simulink subsystem "basic_infeed"  (R2023b)
settings: Solver=VariableStepAuto  StartTime=0.0  StopTime=10.0  RelTol=1e-3
model mask{P=0, Ts=0}
values from neighbouring files (symbols this model uses):
  Ts = ts(k)    [example_MW.m]
libraries: ee_lib x12, fl_lib x4, eeGeneralControl x3, nesl_utility x3, eeTransforms x2, eeSinusoidalMeasurement x1
settings Model: Creator=neugebch  LastModifiedBy=neugebch

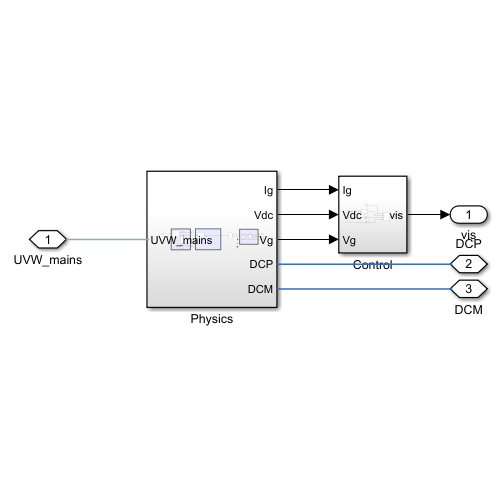
[thumbnail: Simulink's stored preview of the top-level diagram]
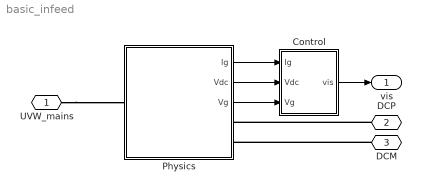
== system basic_infeed ==
  Control : Subsystem
  Physics : Subsystem
  UVW_mains : PMIOPort  Side=Left
  DCP : PMIOPort  Port=2  Side=Right
  DCM : PMIOPort  Port=3  Side=Right
  vis : Outport
  wires:
  Physics/3(Vg) -> Control/3(Vg)
  Physics/2(Vdc) -> Control/2(Vdc)
  Physics/1(Ig) -> Control/1(Ig)
  Control/1(vis) -> vis/1
  connections:
  DCM/RConn1 -- Physics/RConn2
  UVW_mains/RConn1 -- Physics/LConn1
  DCP/RConn1 -- Physics/RConn1

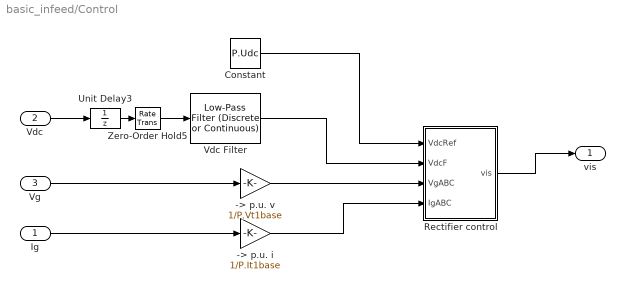
== system basic_infeed/Control ==
  Ig : Inport
  Vdc : Inport  Port=2
  Vg : Inport  Port=3
  -> p.u. i : Gain  Gain=1/P.It1base
  -> p.u. v : Gain  Gain=1/P.Vt1base
  Constant : Constant  Value=P.Udc
  Rectifier control : Subsystem
  Unit Delay3 : UnitDelay  SampleTime=Ts  HasFrameUpgradeWarning=on
  Vdc Filter : eeGeneralControl/Low-Pass Filter (Discrete or Continuous)  K=1  T=1e-3  B=inf  A=-inf  init_option=Inherited from block input  x0=0  Ts=P.Tsc
  Zero-Order Hold5 : RateTransition  OutPortSampleTime=5e-05
  vis : Outport
  wires:
  Zero-Order Hold5/1 -> Vdc Filter/1
  -> p.u. i/1 -> Rectifier control/4(IgABC)
  -> p.u. v/1 -> Rectifier control/3(VgABC)
  Vdc Filter/1 -> Rectifier control/2(VdcF)
  Unit Delay3/1 -> Zero-Order Hold5/1
  Vdc/1 -> Unit Delay3/1
  Constant/1 -> Rectifier control/1(VdcRef)
  Vg/1 -> -> p.u. v/1
  Rectifier control/1(vis) -> vis/1
  Ig/1 -> -> p.u. i/1

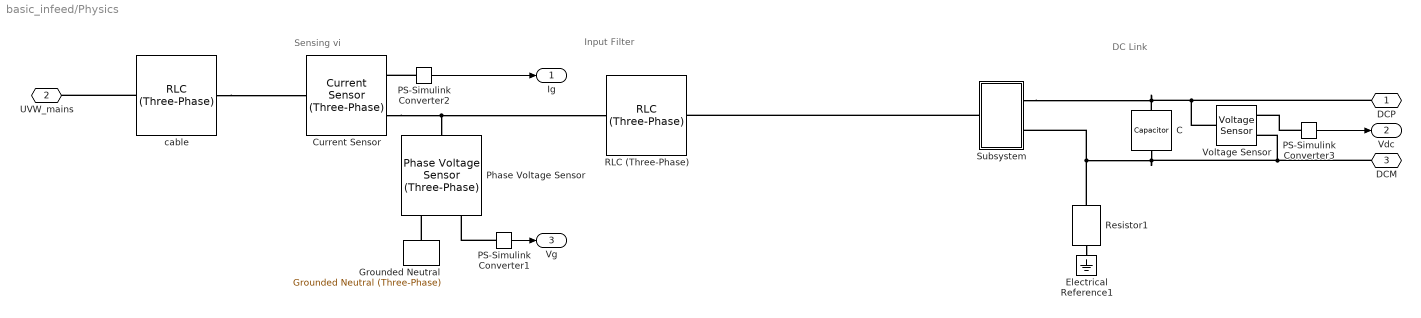
== system basic_infeed/Physics ==
  note: DC
      | Link
  note: Input Filter
  note: Sensing vi
  C : fl_lib/Electrical/Electrical Elements/Capacitor  c=P.Cd F  r=P.Rd Ohm  g=1/P.Rd2 1/Ohm  i_specify=off  i_priority=None  i=0 A  i_nominal_specify=off  i_nominal_unit=A  i_nominal_value=1  v_specify=off  v_priority=None  v=0 V  v_nominal_specify=off  v_nominal_unit=V  v_nominal_value=1  vc_specify=on  vc_priority=None  vc=0 V  vc_nominal_specify=off  vc_nominal_unit=V  vc_nominal_value=1
  Current Sensor : ee_lib/Sensors & Transducers/Current Sensor (Three-Phase)
  Electrical Reference1 : fl_lib/Electrical/Electrical Elements/Electrical Reference
  Grounded Neutral : ee_lib/Connectors & References/Grounded Neutral (Three-Phase)
  PS-Simulink Converter1 : nesl_utility/PS-Simulink Converter  PhysicalDomain=network_engine_domain  SubClassName=ps_output  LeftPortType=input  RightPortType=output  PseudoPeriodic=off  Frequencies=[]  VectorFormat=1-D array  Unit=1  AffineConversion=off
  PS-Simulink Converter2 : nesl_utility/PS-Simulink Converter  PhysicalDomain=network_engine_domain  SubClassName=ps_output  LeftPortType=input  RightPortType=output  PseudoPeriodic=off  Frequencies=[]  VectorFormat=1-D array  Unit=1  AffineConversion=off
  PS-Simulink Converter3 : nesl_utility/PS-Simulink Converter  PhysicalDomain=network_engine_domain  SubClassName=ps_output  LeftPortType=input  RightPortType=output  PseudoPeriodic=off  Frequencies=[]  VectorFormat=1-D array  Unit=1  AffineConversion=off
  Phase Voltage Sensor : ee_lib/Sensors & Transducers/Phase Voltage Sensor (Three-Phase)
  RLC (Three-Phase) : ee_lib/Passive/RLC Assemblies/RLC (Three-Phase)  component_structure=ee.enum.rlc.structure.SeriesRL  R=P.Lk*P.om/P.X_R_Lk Ohm  L=P.Lk H  C=1e-6 F  R_parasitic=0 Ohm  G_parasitic=0 1/Ohm  IL_specify=off  IL_priority=High  IL=[0, 0, 0] A  IL_nominal_specify=off  IL_nominal_unit=A  IL_nominal_value=1  VC_specify=off  VC_priority=High  VC=[0, 0, 0] V  VC_nominal_specify=off  VC_nominal_unit=V  VC_nominal_value=1
      settings: InternalSimscapePortConfiguration="{\"Bottom\":[],\"Left\":[{\"id\":\"N1\",\"label\":\"~1\",\"type\":\"foundation.electrical.three_phase\"}],\"Right\":[{\"id\":\"N2\",\"label\":\"~2\",\"type\":\"foundation.electrical.three_phase\"}],\"Top\":[]}"
  Resistor1 : fl_lib/Electrical/Electrical Elements/Resistor  R=1e5 Ohm  i_specify=off  i_priority=None  i=0 A  i_nominal_specify=off  i_nominal_unit=A  i_nominal_value=1  v_specify=off  v_priority=None  v=0 V  v_nominal_specify=off  v_nominal_unit=V  v_nominal_value=1
  Subsystem : Subsystem
  Voltage Sensor : fl_lib/Electrical/Electrical Sensors/Voltage Sensor
  cable : ee_lib/Passive/RLC Assemblies/RLC (Three-Phase)  component_structure=ee.enum.rlc.structure.SeriesRL  R=P.cab.l*P.cab.rl Ohm  L=P.cab.l*P.cab.ll H  C=1e-6 F  R_parasitic=0 Ohm  G_parasitic=0 1/Ohm  IL_specify=off  IL_priority=High  IL=[0, 0, 0] A  IL_nominal_specify=off  IL_nominal_unit=A  IL_nominal_value=1  VC_specify=off  VC_priority=High  VC=[0, 0, 0] V  VC_nominal_specify=off  VC_nominal_unit=V  VC_nominal_value=1
      settings: InternalSimscapePortConfiguration="{\"Bottom\":[],\"Left\":[{\"id\":\"N1\",\"label\":\"~1\",\"type\":\"foundation.electrical.three_phase\"}],\"Right\":[{\"id\":\"N2\",\"label\":\"~2\",\"type\":\"foundation.electrical.three_phase\"}],\"Top\":[]}"
  DCP : PMIOPort  Side=Right
  UVW_mains : PMIOPort  Port=2  Side=Left
  DCM : PMIOPort  Port=3  Side=Right
  Ig : Outport
  Vdc : Outport  Port=2
  Vg : Outport  Port=3
  wires:
  PS-Simulink Converter1/1 -> Vg/1
  PS-Simulink Converter2/1 -> Ig/1
  PS-Simulink Converter3/1 -> Vdc/1
  connections:
  cable/RConn1 -- Current Sensor/LConn1
  cable/LConn1 -- UVW_mains/RConn1
  Subsystem/LConn1 -- RLC (Three-Phase)/RConn1
  PS-Simulink Converter1/LConn1 -- Phase Voltage Sensor/RConn1
  Grounded Neutral/LConn1 -- Phase Voltage Sensor/RConn2
  Subsystem/RConn2 -- DCM/RConn1 -- Voltage Sensor/RConn2 -- C/RConn1 -- Resistor1/LConn1
  PS-Simulink Converter2/LConn1 -- Current Sensor/RConn1
  Current Sensor/RConn2 -- RLC (Three-Phase)/LConn1 -- Phase Voltage Sensor/LConn1
  C/LConn1 -- Subsystem/RConn1 -- Voltage Sensor/LConn1 -- DCP/RConn1
  PS-Simulink Converter3/LConn1 -- Voltage Sensor/RConn1
  Resistor1/RConn1 -- Electrical Reference1/LConn1

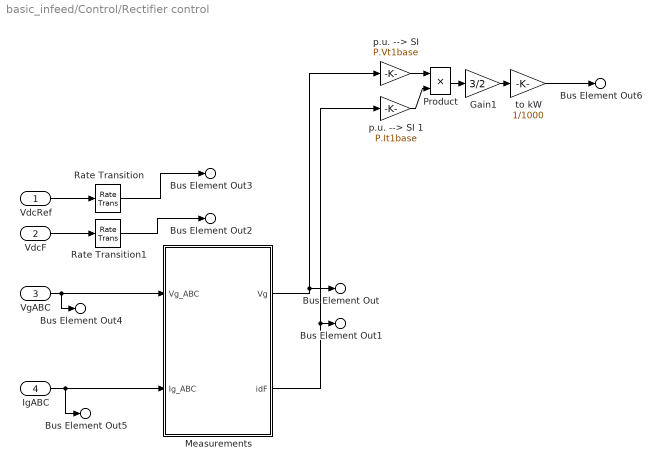
== system basic_infeed/Control/Rectifier control ==
  VdcRef : Inport
  VdcF : Inport  Port=2
  VgABC : Inport  Port=3
  IgABC : Inport  Port=4
  Gain1 : Gain  Gain=3/2
  Measurements : Subsystem
  Product : Product
  Rate Transition : RateTransition
  Rate Transition1 : RateTransition
  p.u. --> SI : Gain  Gain=P.Vt1base
  p.u. --> SI 1 : Gain  Gain=P.It1base
  to kW : Gain  Gain=1/1000
  Bus Element Out : Outport  PortName=vis  Element=Vg
  Bus Element Out1 : Outport  PortName=vis  Element=idF
  Bus Element Out2 : Outport  PortName=vis  Element=VdcF
  Bus Element Out3 : Outport  PortName=vis  Element=VdcRef
  Bus Element Out4 : Outport  PortName=vis  Element=VgABC
  Bus Element Out5 : Outport  PortName=vis  Element=IgABC
  Bus Element Out6 : Outport  PortName=vis  Element=Pt
  wires:
  VdcRef/1 -> Rate Transition/1
  VdcF/1 -> Rate Transition1/1
  VgABC/1 -> Bus Element Out4/1, Measurements/1(Vg_ABC)
  IgABC/1 -> Bus Element Out5/1, Measurements/2(Ig_ABC)
  Rate Transition/1 -> Bus Element Out3/1
  Rate Transition1/1 -> Bus Element Out2/1
  Measurements/1(Vg) -> p.u. --> SI/1, Bus Element Out/1
  Product/1 -> Gain1/1
  p.u. --> SI 1/1 -> Product/2
  p.u. --> SI/1 -> Product/1
  Gain1/1 -> to kW/1
  Measurements/2(idF) -> p.u. --> SI 1/1, Bus Element Out1/1
  to kW/1 -> Bus Element Out6/1

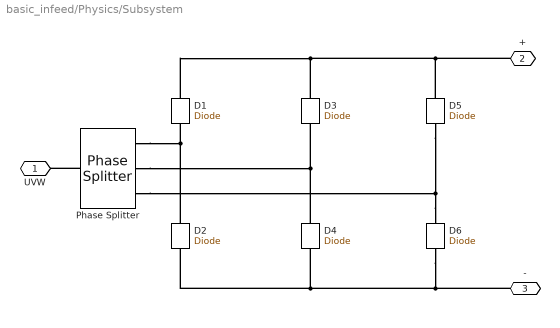
== system basic_infeed/Physics/Subsystem ==
  D{1..6} (6 alike) : ee_lib/Semiconductors & Converters/Diode  ModelType=ee.enum.diode.modelType.pwl  TableType=ee.enum.diode.tableType.IfMat  IfMat=[.07, .12, .19, 1.75, 4.24, 7.32, 11.2; .16, .3, .72, 2.14, 4.02, 6.35, 9.12] A  VfMat=[.9, 1.15, 1.25, 1.5, 1.75, 2.17, 2.6, 2.85; .58, .68, .75, 1.1, 1.38, 1.77, 2.27, 2.7] V  TjVec=[25, 125] degC  VfVec=[.5, .7, .9, 1.3, 1.7, 2.1, 2.5] V  IfVec=[.1, .2, .5, 1, 2, 4, 7, 10] A  Vf=0.6 V  Ron=0.3 Ohm  Goff=1e-8 S  prmExp=2  I12=[ 0.0137 0.545 ] A  V12=[ 0.6 0.7 ] V  RS=0.001 Ohm  Tmeas=25 degC  IS=1e-7 A  ec=1  I1=0.0137 A  V1=0.6 V  N_series=1  N_parallel=1  ZenerEnable=false  Rz=0.3 Ohm  BV=Inf V  C_param=1  CJ=50 pF  CJ0=50 pF  Vvec=[ 0.1 10 100 ] V  Cvec=[ 3.5 1 0.4 ] pF  VJ=1 V  Mgrad=0.5  FC=0.5  Q_param=ee.enum.diode.recoveryParam.off  iRM=-7.15 A  iF=4 A  didt=-750 A/us  trr_factor=3  trr=115 ns  Qrr=1500 s*uA  Vr=-600 V  Ls=150 nH  Erec=0.03 J  TT=50 ns  tau=100 ns  T_param=1  Tdevice=25 degC  I1_T2=0.245 A  V1_T2=0.5 V  IS_T2=1.25e-7 A  Tmeas2=125 degC  XTI_param=1  XTI=3  EG_param=1  EG=1.11 eV  dBVdT=0 V/K  enable_faults=ee.enum.enable.no  fault_action=simscape.enum.assert.action.none  fault_types=ee.enum.diode.faults.open  tau_fault=1e-3 s  IfMat_faulted=[.07, .12, .19, 1.75, 4.24, 7.32, 11.2; .16, .3, .72, 2.14, 4.02, 6.35, 9.12] A  VfMat_faulted=[.9, 1.15, 1.25, 1.5, 1.75, 2.17, 2.6, 2.85; .58, .68, .75, 1.1, 1.38, 1.77, 2.27, 2.7] V  VfVec_faulted=[.5, .7, .9, 1.3, 1.7, 2.1, 2.5] V  IfVec_faulted=[.1, .2, .5, 1, 2, 4, 7, 10] A  Ropen_faulted=1000 Ohm  Gshort_faulted=1000 1/Ohm  Vf_faulted=0.6 V  Ron_faulted=0.3 Ohm  Goff_faulted=1e-8 S  I12_faulted=[.0137, .545] A  V12_faulted=[.6, .7] V  IS_faulted=1e-12 A  ec_faulted=1  I1_faulted=0.0137 A  V1_faulted=0.6 V  RS_faulted=0 Ohm  Rz_faulted=0.3 Ohm  BV_faulted=inf V  Cscale_faulted=100  fault_trigger=ee.enum.faults.faultTrigger.temporal  t_fault=inf s  max_permissible_voltage=inf V  n_fail_on_voltage=1  max_permissible_current=inf A  t_fail_on_current=1 s  max_permissible_dVdt=inf V/s  enable_fault_input=simscape.enum.onoff.off  i_specify=off  i_priority=None  i=0 A  i_nominal_specify=off  i_nominal_unit=A  i_nominal_value=1  v_specify=off  v_priority=None  v=0 V  v_nominal_specify=off  v_nominal_unit=V  v_nominal_value=1  v_capacitor_specify=off  v_capacitor_priority=None  v_capacitor=0 V  v_capacitor_nominal_specify=off  v_capacitor_nominal_unit=V  v_capacitor_nominal_value=1  faulted_specify=off  faulted_priority=None  faulted=0  faulted_nominal_specify=off  faulted_nominal_unit=1  faulted_nominal_value=1  i_diode_specify=off  i_diode_priority=None  i_diode=0 A  i_diode_nominal_specify=off  i_diode_nominal_unit=A  i_diode_nominal_value=1  v_diode_specify=off  v_diode_priority=None  v_diode=0 V  v_diode_nominal_specify=off  v_diode_nominal_unit=V  v_diode_nominal_value=1  i_capacitor_specify=off  i_capacitor_priority=High  i_capacitor=0 A  i_capacitor_nominal_specify=off  i_capacitor_nominal_unit=A  i_capacitor_nominal_value=1  power_dissipated_specify=off  power_dissipated_priority=None  power_dissipated=0 W  power_dissipated_nominal_specify=off  power_dissipated_nominal_unit=W  power_dissipated_nominal_value=1  fidelity_level=ee.enum.diode.fidelity.includeChargeDyn  rec_loss_model=ee.enum.diode.reverseRecoveryModel.fixed  ErecVal=0 J  scaleWithIandV=true  ErecMat=zeros(2, 3) J  TjrecVec=[298.15, 398.15] K  IfrecVec=[.1, 1, 10] A  IrecVal=10 A  VrecVal=10 V  tFilter=1 / 1000 / 100 s  max_permissible_temperature=inf K  t_fail_on_temperature=1 s  thermal_network_parameterization=ee.enum.thermalNetworkTopology.junctionCase  Rth=[0, 10] K/W  Rth_Cauer=[1, 3, 10] K/W  Rth_Foster=[4, 6] K/W  thermal_mass_parameterization=ee.enum.thermalNetwork.timeconstant  thermal_mass=[0, 1] J/K  thermal_mass_Cauer=[.1, .3, 1] J/K  thermal_mass_Foster=[1.5, 3] J/K  thermal_time_constant=[0, 10] s  thermal_time_constant_Cauer=[1, 3, 10] s  thermal_time_constant_Foster=[6, 18] s  thermal_mass_initial_temperatures=[25, 25] degC  thermal_mass_initial_temperatures_Cauer=[25, 25, 25] degC  junction_thermal_mass=0.01 J/K  Tvec_initial_Foster=[25, 25, 25, 25] degC  no_thermal_network=0  junction_temperature_specify=off  junction_temperature_priority=None  junction_temperature=25 degC  junction_temperature_nominal_specify=off  junction_temperature_nominal_unit=degC  junction_temperature_nominal_value=1
      settings: LogSimulationData=on
  Phase Splitter : ee_lib/Connectors & References/Phase Splitter
  UVW : PMIOPort  Side=Left
  + : PMIOPort  Tag=PMCPort  Port=2  Side=Right
  - : PMIOPort  Tag=PMCPort  Port=3  Side=Right
  connections:
  Phase Splitter/LConn1 -- UVW/RConn1
  D2/LConn1 -- D6/LConn1 -- -/RConn1 -- D4/LConn1
  D6/RConn1 -- Phase Splitter/RConn3 -- D5/LConn1
  D1/LConn1 -- Phase Splitter/RConn1 -- D2/RConn1
  D4/RConn1 -- Phase Splitter/RConn2 -- D3/LConn1
  D3/RConn1 -- D5/RConn1 -- +/RConn1 -- D1/RConn1

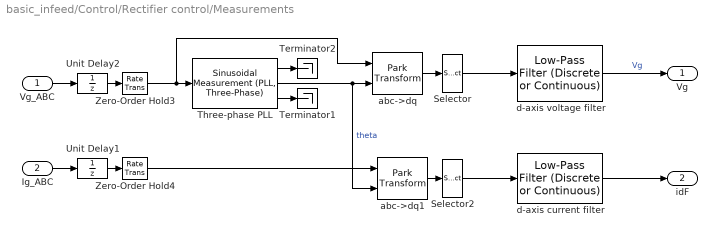
== system basic_infeed/Control/Rectifier control/Measurements ==
  Vg_ABC : Inport
  Ig_ABC : Inport  Port=2
  Selector : Selector  InputPortWidth=3  IndexOptions=Index vector (dialog)  Indices=[1]  OutputSizes=1
  Selector2 : Selector  InputPortWidth=3  IndexOptions=Index vector (dialog)  Indices=[1]  OutputSizes=1
  Terminator1 : Terminator
  Terminator2 : Terminator
  Three-phase PLL : eeSinusoidalMeasurement/Sinusoidal Measurement (PLL, Three-Phase)  Kp_LF=45  Ki_LF=1250  F0=fn  Theta0=0  Ts=P.Tsc
  Unit Delay1 : UnitDelay  SampleTime=Ts  HasFrameUpgradeWarning=on
  Unit Delay2 : UnitDelay  SampleTime=Ts  HasFrameUpgradeWarning=on
  Zero-Order Hold3 : RateTransition  OutPortSampleTime=5e-05
  Zero-Order Hold4 : RateTransition  OutPortSampleTime=5e-05
  abc->dq : eeTransforms/Park Transform  AxisAlignment=Q-axis  PowerInvariant=off
  abc->dq1 : eeTransforms/Park Transform  AxisAlignment=Q-axis  PowerInvariant=off
  d-axis current filter : eeGeneralControl/Low-Pass Filter (Discrete or Continuous)  K=1  T=1e-3  B=inf  A=-inf  init_option=Inherited from block input  x0=0  Ts=P.Tsc
  d-axis voltage filter : eeGeneralControl/Low-Pass Filter (Discrete or Continuous)  K=1  T=1e-3  B=inf  A=-inf  init_option=Inherited from block input  x0=0  Ts=P.Tsc
  Vg : Outport  VectorParamsAs1DForOutWhenUnconnected=off
  idF : Outport  Port=2  VectorParamsAs1DForOutWhenUnconnected=off
  wires:
  Three-phase PLL/1 -> Terminator2/1
  Selector2/1 -> d-axis current filter/1
  Unit Delay1/1 -> Zero-Order Hold4/1
  abc->dq/1 -> Selector/1
  Three-phase PLL/2 -> abc->dq1/2, abc->dq/2  "theta"
  d-axis current filter/1 -> idF/1
  Zero-Order Hold3/1 -> abc->dq/1, Three-phase PLL/1
  Selector/1 -> d-axis voltage filter/1
  Three-phase PLL/3 -> Terminator1/1
  Ig_ABC/1 -> Unit Delay1/1
  d-axis voltage filter/1 -> Vg/1  "Vg"
  Zero-Order Hold4/1 -> abc->dq1/1
  Unit Delay2/1 -> Zero-Order Hold3/1
  abc->dq1/1 -> Selector2/1
  Vg_ABC/1 -> Unit Delay2/1
